simulink model "Examples"  (R2022b)
settings: Solver=daessc  StartTime=0.0  StopTime=1.0  MaxStep=1e-4  RelTol=1e-3  AbsTol=1e-3
InitFcn:
  | load('vars')
undefined symbols (not defined in the file): D_0, K_0, Re
libraries: nesl_utility x9, acoustical_lib x8, fl_lib x6, SpeakerSubsystemLibrary_1_0_0 x2, simulink x1
settings Model: Creator=sct12  LastModifiedBy=sct12
settings SolverCC: AutoScaleAbsTol=off  AlgebraicLoopSolver=TrustRegion  MaxZcPerStep=1
settings DebuggingCC: UnconnectedInputMsg=warning  UnconnectedOutputMsg=warning  UnconnectedLineMsg=warning  SymbolicDimsDataTypeCodeGenerationDiagnostic=none  SFMachineParentedDataDiag=warning
settings ModelReferenceCC: EnableRefExpFcnMdlSchedulingChecks=on
settings SFSimCC: CustomCodeUndefinedFunction=UseInterfaceOnly
settings RTWCC: DLArmComputeVersion=19.05
settings SimscapeCC: SimscapeLogType=all  SimscapeLogSimulationStatistics=on  SimscapeLogDataHistory=10000

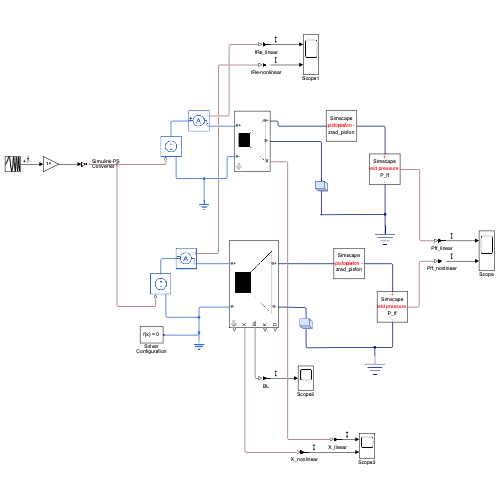
[thumbnail: Simulink's stored preview of the top-level diagram]
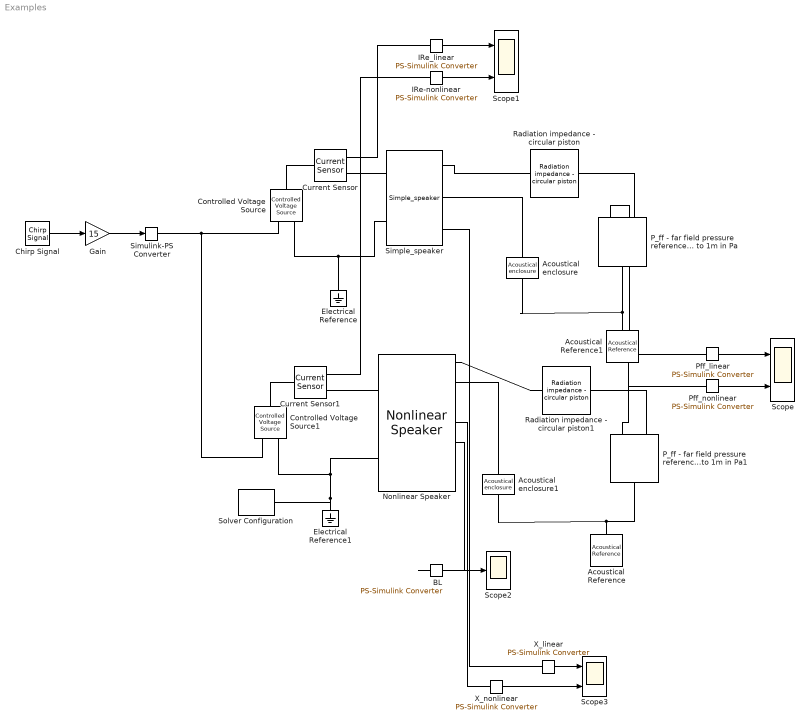
== system Examples ==
  Acoustical Reference : acoustical_lib/Acoustical Elements/Acoustical Reference
      settings: SourceProductName=Acoustical  InternalSimscapePortConfiguration="{\"Bottom\":[],\"Left\":[{\"id\":\"pp\",\"label\":\"\",\"type\":\"acoustical.acoustical\"}],\"Right\":[],\"Top\":[]}"
  Acoustical Reference1 : acoustical_lib/Acoustical Elements/Acoustical Reference
      settings: SourceProductName=Acoustical  InternalSimscapePortConfiguration="{\"Bottom\":[],\"Left\":[{\"id\":\"pp\",\"label\":\"\",\"type\":\"acoustical.acoustical\"}],\"Right\":[],\"Top\":[]}"
  Acoustical enclosure : acoustical_lib/Acoustical Elements/Acoustical enclosure  vol=1.5 l
      settings: SourceProductName=Acoustical  InternalSimscapePortConfiguration="{\"Bottom\":[],\"Left\":[{\"id\":\"pp\",\"label\":\"+\",\"type\":\"acoustical.acoustical\"}],\"Right\":[{\"id\":\"nn\",\"label\":\"-\",\"type\":\"acoustical.acoustical\"}],\"Top\":[]}"
  Acoustical enclosure1 : acoustical_lib/Acoustical Elements/Acoustical enclosure  vol=1.5 l
      settings: SourceProductName=Acoustical  InternalSimscapePortConfiguration="{\"Bottom\":[],\"Left\":[{\"id\":\"pp\",\"label\":\"+\",\"type\":\"acoustical.acoustical\"}],\"Right\":[{\"id\":\"nn\",\"label\":\"-\",\"type\":\"acoustical.acoustical\"}],\"Top\":[]}"
  BL : nesl_utility/PS-Simulink Converter  PhysicalDomain=network_engine_domain  SubClassName=ps_output  LeftPortType=input  RightPortType=output  PseudoPeriodic=off  Frequencies=[]  VectorFormat=inherit  Unit=inherit  AffineConversion=off
  Chirp Signal : simulink/Sources/Chirp Signal  f1=50  T=10  f2=50
  Controlled Voltage Source : fl_lib/Electrical/Electrical Sources/Controlled Voltage Source
  Controlled Voltage Source1 : fl_lib/Electrical/Electrical Sources/Controlled Voltage Source
  Current Sensor : fl_lib/Electrical/Electrical Sensors/Current Sensor
  Current Sensor1 : fl_lib/Electrical/Electrical Sensors/Current Sensor
  Electrical Reference : fl_lib/Electrical/Electrical Elements/Electrical Reference
  Electrical Reference1 : fl_lib/Electrical/Electrical Elements/Electrical Reference
  Gain : Gain  Gain=15
  IRe-nonlinear : nesl_utility/PS-Simulink Converter  PhysicalDomain=network_engine_domain  SubClassName=ps_output  LeftPortType=input  RightPortType=output  PseudoPeriodic=off  Frequencies=[]  VectorFormat=inherit  Unit=inherit  AffineConversion=off
  IRe_linear : nesl_utility/PS-Simulink Converter  PhysicalDomain=network_engine_domain  SubClassName=ps_output  LeftPortType=input  RightPortType=output  PseudoPeriodic=off  Frequencies=[]  VectorFormat=inherit  Unit=inherit  AffineConversion=off
  Nonlinear Speaker : SpeakerSubsystemLibrary_1_0_0/Nonlinear Speaker  Sd=Sd m^2  mass=Mm kg  R=Re Ohm  L2=L2 H  R2=R2 Ohm  L0_of_x=Le_0 H  L1_of_x=Le_1 H/m  L2_of_x=Le_2 H/m^2  L3_of_x=Le_3 H/m^3  L4_of_x=Le_4 H/m^4  Bl0=BL_0 N/A  Bl1=BL_1 N/(A*m)  Bl2=BL_2 N/(A*m^2)  Bl3=BL_3 N/(A*m^3)  Bl4=BL_4 N/(A*m^4)  K0=K_0 N/m  K1=K_1 N/m^2  K2=K_2 N/m^3  K3=K_3 N/m^4  K4=K_4 N/m^5  D0=D_0 N*s/m  D1=D_1 N*s^2/m^2  D2=D_2 N*s^3/m^3  D3=D_3 N*s^4/m^4  D4=D_4 N*s^5/m^5
  P_ff - far field pressure referenced to 1m in Pa : acoustical_lib/Acoustical Elements/P_ff - far field pressure referenced to 1m in Pa  dist=1 m  u_specify=off  u_priority=None  u=0 m^3/s  u_nominal_specify=off  u_nominal_unit=m^3/s  u_nominal_value=1  p_specify=off  p_priority=None  p=0 Pa  p_nominal_specify=off  p_nominal_unit=Pa  p_nominal_value=1
      settings: SourceProductName=Acoustical  InternalSimscapePortConfiguration="{\"Bottom\":[],\"Left\":[{\"id\":\"pp\",\"label\":\"+\",\"type\":\"acoustical.acoustical\"}],\"Right\":[{\"id\":\"nn\",\"label\":\"-\",\"type\":\"acoustical.acoustical\"}],\"Top\":[{\"id\":\"p_ff\",\"label\":\"far field pressure\",\"type\":\"output\"}]}"
  P_ff - far field pressure referenced to 1m in Pa1 : acoustical_lib/Acoustical Elements/P_ff - far field pressure referenced to 1m in Pa  dist=1 m  u_specify=off  u_priority=None  u=0 m^3/s  u_nominal_specify=off  u_nominal_unit=m^3/s  u_nominal_value=1  p_specify=off  p_priority=None  p=0 Pa  p_nominal_specify=off  p_nominal_unit=Pa  p_nominal_value=1
      settings: SourceProductName=Acoustical  InternalSimscapePortConfiguration="{\"Bottom\":[],\"Left\":[{\"id\":\"pp\",\"label\":\"+\",\"type\":\"acoustical.acoustical\"}],\"Right\":[{\"id\":\"nn\",\"label\":\"-\",\"type\":\"acoustical.acoustical\"}],\"Top\":[{\"id\":\"p_ff\",\"label\":\"far field pressure\",\"type\":\"output\"}]}"
  Pff_linear : nesl_utility/PS-Simulink Converter  PhysicalDomain=network_engine_domain  SubClassName=ps_output  LeftPortType=input  RightPortType=output  PseudoPeriodic=off  Frequencies=[]  VectorFormat=inherit  Unit=inherit  AffineConversion=off
  Pff_nonlinear : nesl_utility/PS-Simulink Converter  PhysicalDomain=network_engine_domain  SubClassName=ps_output  LeftPortType=input  RightPortType=output  PseudoPeriodic=off  Frequencies=[]  VectorFormat=inherit  Unit=inherit  AffineConversion=off
  Radiation impedance - circular piston : acoustical_lib/Acoustical Elements/Radiation impedance - circular piston  Sd=Sd m^2
      settings: SourceProductName=Acoustical  InternalSimscapePortConfiguration="{\"Bottom\":[],\"Left\":[{\"id\":\"pa\",\"label\":\"piston +\",\"type\":\"acoustical.acoustical\"}],\"Right\":[{\"id\":\"na\",\"label\":\"piston -\",\"type\":\"acoustical.acoustical\"}],\"Top\":[]}"
  Radiation impedance - circular piston1 : acoustical_lib/Acoustical Elements/Radiation impedance - circular piston  Sd=Sd m^2
      settings: SourceProductName=Acoustical  InternalSimscapePortConfiguration="{\"Bottom\":[],\"Left\":[{\"id\":\"pa\",\"label\":\"piston +\",\"type\":\"acoustical.acoustical\"}],\"Right\":[{\"id\":\"na\",\"label\":\"piston -\",\"type\":\"acoustical.acoustical\"}],\"Top\":[]}"
  Scope : Scope  NumInputPorts=2
  Scope1 : Scope  NumInputPorts=2
  Scope2 : Scope
  Scope3 : Scope  NumInputPorts=2
  Simple_speaker : SpeakerSubsystemLibrary_1_0_0/Simple_speaker  Re=Re Ohm  Le=Le_0 H  L2=L2 H  R2=R2 Ohm  BL=BL_0 V*s/m  Mm=Mm kg  K=K_0 N/m  D=D_0 N*s/m  Sd=Sd m^2
  Simulink-PS Converter : nesl_utility/Simulink-PS Converter  PhysicalDomain=network_engine_domain  SubClassName=ps_input  LeftPortType=input  RightPortType=output  PseudoPeriodic=off  Frequencies=[]  NoiseDistribution=none  NoiseParameters=[]  Unit=1  AffineConversion=off  FilteringAndDerivatives=filter  SimscapeFilterOrder=1  InputFilterTimeConstant=0.000001  UdotUserProvided=0
  Solver Configuration : nesl_utility/Solver Configuration  PhysicalDomain=network_engine_domain  SubClassName=solver  LeftPortType=input  RightPortType=generic  Tones=[]  Harmonics=[]  SimulateNoise=off  Profile=off  UseLocalSampling=off  EnableSwitchedLinearOptims=on  FrequencyDomain=off  UseCCode=off  RelTol=0.001  AbsTol=1e-06  MinStep=1e-09  ToWorkspace=off  RevertToSquareIcSolve=off  NumHomotopyIterations=100  PhasorMode=off  PhasorModeNumHarmonics=1  ConsistencySolver=NEWTON_XTOL_AFTER_FTOL  IndexReductionMethod=DerivativeReplacement  DoDC=off  ResidualTolerance=1e-09  ConsistencyTolSource=GLOBAL  ConsistencyAbsTol=0.001  ConsistencyRelTol=0.001  ConsistencyTolFactor=0.001  UseLocalSolver=off  LocalSolverChoice=NE_BACKWARD_EULER_ADVANCER  ResolveIndetEquations=on  FunctionEvalNumThread=1  LocalSolverSampleTime=0.001  DoFixedCost=off  MaxNonlinIter=3  MaxModeIter=2  ComputeImpulses=off  ImpulseIterations=2  LinearAlgebra=auto  LinearAlgebraNumThread=0  EquationFormulation=NE_TIME_EF  DelaysMemoryBudget=1024  AutomaticFiltering=on  FilteringTimeConstant=0.001  PartitionStorageMethod=AS_NEEDED  PartitionMemoryBudget=1024  PartitionMethod=ROBUST
  X_linear : nesl_utility/PS-Simulink Converter  PhysicalDomain=network_engine_domain  SubClassName=ps_output  LeftPortType=input  RightPortType=output  PseudoPeriodic=off  Frequencies=[]  VectorFormat=inherit  Unit=inherit  AffineConversion=off
  X_nonlinear : nesl_utility/PS-Simulink Converter  PhysicalDomain=network_engine_domain  SubClassName=ps_output  LeftPortType=input  RightPortType=output  PseudoPeriodic=off  Frequencies=[]  VectorFormat=inherit  Unit=inherit  AffineConversion=off
  wires:
  Pff_linear/1 -> Scope/1
  Pff_nonlinear/1 -> Scope/2
  Chirp Signal/1 -> Gain/1
  IRe_linear/1 -> Scope1/1
  IRe-nonlinear/1 -> Scope1/2
  Gain/1 -> Simulink-PS Converter/1
  BL/1 -> Scope2/1
  X_nonlinear/1 -> Scope3/2
  X_linear/1 -> Scope3/1
  connections:
  Radiation impedance - circular piston/LConn1 -- Simple_speaker/RConn1
  P_ff - far field pressure referenced to 1m in Pa/LConn1 -- Radiation impedance - circular piston/RConn1
  P_ff - far field pressure referenced to 1m in Pa/LConn2 -- Pff_linear/LConn1
  P_ff - far field pressure referenced to 1m in Pa1/LConn1 -- Radiation impedance - circular piston1/RConn1
  Acoustical Reference/LConn1 -- P_ff - far field pressure referenced to 1m in Pa1/RConn1 -- Acoustical enclosure1/RConn1
  Radiation impedance - circular piston1/LConn1 -- Nonlinear Speaker/RConn1
  Acoustical Reference1/LConn1 -- Acoustical enclosure/RConn1 -- P_ff - far field pressure referenced to 1m in Pa/RConn1
  Nonlinear Speaker/LConn1 -- Current Sensor1/RConn2
  Controlled Voltage Source1/LConn1 -- Current Sensor1/LConn1
  Current Sensor/LConn1 -- Controlled Voltage Source/LConn1
  Controlled Voltage Source/RConn2 -- Electrical Reference/LConn1 -- Simple_speaker/LConn2
  Controlled Voltage Source1/RConn2 -- Nonlinear Speaker/LConn2 -- Solver Configuration/RConn1 -- Electrical Reference1/LConn1
  Controlled Voltage Source/RConn1 -- Controlled Voltage Source1/RConn1 -- Simulink-PS Converter/RConn1
  P_ff - far field pressure referenced to 1m in Pa1/LConn2 -- Pff_nonlinear/LConn1
  Current Sensor/RConn2 -- Simple_speaker/LConn1
  IRe_linear/LConn1 -- Current Sensor/RConn1
  IRe-nonlinear/LConn1 -- Current Sensor1/RConn1
  Simple_speaker/RConn2 -- Acoustical enclosure/LConn1
  Acoustical enclosure1/LConn1 -- Nonlinear Speaker/RConn2
  BL/LConn1 -- Nonlinear Speaker/RConn5
  Nonlinear Speaker/RConn4 -- X_nonlinear/LConn1
  X_linear/LConn1 -- Simple_speaker/RConn3
